simulink model "DisplayModel_Step2_start"  (R2013b)
settings: Solver=FixedStepDiscrete  StartTime=0.0  StopTime=10.0  FixedStep=0.2  RelTol=1e-3
undefined symbols (not defined in the file): sigbuilder_block
libraries: simulink x6
settings Model: CovHTMLOptions=-sRT=1 -aTS=1 -bRG=1 -bTC=1 -hTR=0 -nFC=0 -scm=1 -bcm=1 -xEv=0  Creator=siddhars  LastModifiedBy=rruff
settings OptimizationCC: ExpressionDepthLimit=2147483647
settings DebuggingCC: StateNameClashWarn=warning

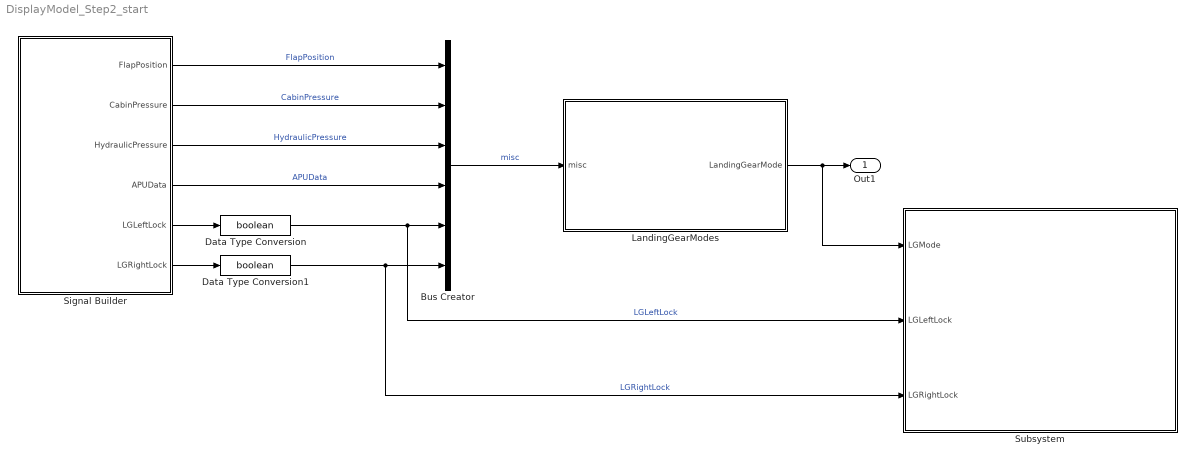
== system DisplayModel_Step2_start ==
  Bus Creator : BusCreator  Inputs=6  OutDataTypeStr=Bus: MiscData
  Data Type Conversion : DataTypeConversion  OutDataTypeStr=boolean
  Data Type Conversion1 : DataTypeConversion  OutDataTypeStr=boolean
  LandingGearModes : Stateflow chart  TreatAsAtomicUnit=on
  Signal Builder : Subsystem  Tag=STV Subsys  LoadFcn=sigbuilder_block('load');  StartFcn=sigbuilder_block('start');  StopFcn=sigbuilder_block('stop');  ClipboardFcn=sigbuilder_block('clipboard');  mask(Sigbuilder block){}
      mask help: Simulink:masks:SigbuilderBlock_MD
      mask init:
      | if ~strcmp(get_param(bdroot(gcbh),'SimulationStatus'),'stopped') tuvar = sigbuilder_block('maskInit'); end
      settings: CopyFcn=sigbuilder_block('copy');  DeleteFcn=sigbuilder_block('delete');  ModelCloseFcn=sigbuilder_block('modelClose');  PreSaveFcn=sigbuilder_block('preSave');  PauseFcn=sigbuilder_block('pause');  ContinueFcn=sigbuilder_block('continue');  NameChangeFcn=sigbuilder_block('namechange');  OpenFcn=sigbuilder_block('open',[43.5 185.25 692.25 402.75 ]);  CloseFcn=sigbuilder_block('close');
      mask Display: plot(0, 0, 100, 100,[2, 2, 32, 32, 2], [68, 8, 8, 68, 68],[32, 2], [38, 38], [32, 19, 2],[53, 60, 44], [32, 17, 17, 2],[16, 16, 31, 31]);txt = getActiveGroup(gcbh);text(2, 100, txt,'verticalAlignment', 'top');
  Subsystem : Subsystem
  Out1 : Outport
  wires:
  LandingGearModes/1(LandingGearMode) -> Subsystem/1(LGMode), Out1/1
  Signal Builder/6(LGRightLock) -> Data Type Conversion1/1
  Signal Builder/5(LGLeftLock) -> Data Type Conversion/1
  Data Type Conversion1/1 -> Subsystem/3(LGRightLock), Bus Creator/6  "LGRightLock"
  Data Type Conversion/1 -> Subsystem/2(LGLeftLock), Bus Creator/5  "LGLeftLock"
  Signal Builder/1(FlapPosition) -> Bus Creator/1  "FlapPosition"
  Signal Builder/3(HydraulicPressure) -> Bus Creator/3  "HydraulicPressure"
  Signal Builder/4(APUData) -> Bus Creator/4  "APUData"
  Signal Builder/2(CabinPressure) -> Bus Creator/2  "CabinPressure"
  Bus Creator/1 -> LandingGearModes/1(misc)  "misc"

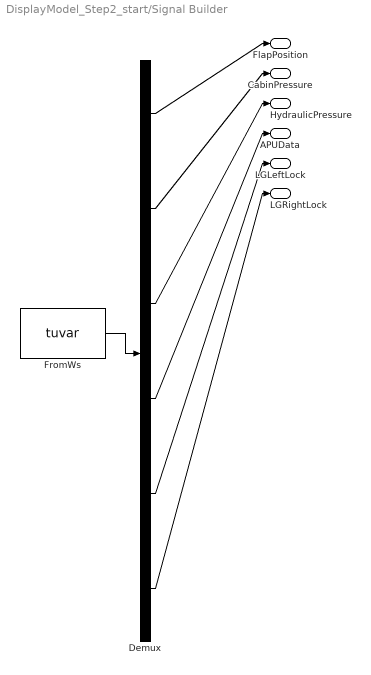
== system DisplayModel_Step2_start/Signal Builder ==
  Demux : Demux  Tag=STV Demux  Outputs=6
  FromWs : FromWorkspace  Tag=STV FromWs  VariableName=tuvar  SampleTime=0
      SigBuilderData=|
      | common.afterFinalStr = 'Extrapolate'
      | common.sampleTime = 0
      | dataSet(1).timeRange = [0 10]
      | dataSet(1).name = 'BothOn'
      | dataSet(2).timeRange = [0 10]
      | dataSet(2).name = 'OneOnA'
      | dataSet(3).timeRange = [0 10]
      | dataSet(3).name = 'OneOnB'
      | dataSet(4).timeRange = [0 10]
      | dataSet(4).name = 'BothOFF'
      | sbobj.Groups(1).Name = 'BothOn'
      | sbobj.Groups(1).Signals(1).Name = 'FlapPosition'
      | sbobj.Groups(1).Signals(1).XData = [0 10]
      | sbobj.Groups(1).Signals(1).YData = [0 0]
      | sbobj.Groups(1).Signals(2).Name = 'CabinPressure'
      | sbobj.Groups(1).Signals(2).XData = [0 10]
      | sbobj.Groups(1).Signals(2).YData = [0 0]
      | sbobj.Groups(1).Signals(3).Name = 'HydraulicPressure'
      | sbobj.Groups(1).Signals(3).XData = [0 10]
      | sbobj.Groups(1).Signals(3).YData = [0 0]
      | sbobj.Groups(1).Signals(4).Name = 'APUData'
      | sbobj.Groups(1).Signals(4).XData = [0 10]
      | sbobj.Groups(1).Signals(4).YData = [0 0]
      | sbobj.Groups(1).Signals(5).Name = 'LGLeftLock'
      | sbobj.Groups(1).Signals(5).XData = [0 1.74 6.62 10]
      | sbobj.Groups(1).Signals(5).YData = [1 1 1 1]
      | sbobj.Groups(1).Signals(6).Name = 'LGRightLock'
      | sbobj.Groups(1).Signals(6).XData = [0 3.36 7.8 10]
      | sbobj.Groups(1).Signals(6).YData = [1 1 1 1]
      | sbobj.Groups(2).Name = 'OneOnA'
      | sbobj.Groups(2).Signals(1).Name = 'FlapPosition'
      | sbobj.Groups(2).Signals(1).XData = [0 10]
      | sbobj.Groups(2).Signals(1).YData = [0 0]
      | sbobj.Groups(2).Signals(2).Name = 'CabinPressure'
      | sbobj.Groups(2).Signals(2).XData = [0 10]
      | sbobj.Groups(2).Signals(2).YData = [0 0]
      | sbobj.Groups(2).Signals(3).Name = 'HydraulicPressure'
      | sbobj.Groups(2).Signals(3).XData = [0 10]
      | sbobj.Groups(2).Signals(3).YData = [0 0]
      | sbobj.Groups(2).Signals(4).Name = 'APUData'
      | sbobj.Groups(2).Signals(4).XData = [0 10]
      | sbobj.Groups(2).Signals(4).YData = [0 0]
      | sbobj.Groups(2).Signals(5).Name = 'LGLeftLock'
      | sbobj.Groups(2).Signals(5).XData = [0 5.02 5.02 10]
      | sbobj.Groups(2).Signals(5).YData = [1 1 0 0]
      | sbobj.Groups(2).Signals(6).Name = 'LGRightLock'
      | sbobj.Groups(2).Signals(6).XData = [0 5.02 5.02 10]
      | sbobj.Groups(2).Signals(6).YData = [0 0 1 1]
      | sbobj.Groups(3).Name = 'OneOnB'
      | sbobj.Groups(3).Signals(1).Name = 'FlapPosition'
      | sbobj.Groups(3).Signals(1).XData = [0 10]
      | sbobj.Groups(3).Signals(1).YData = [0 0]
      | sbobj.Groups(3).Signals(2).Name = 'CabinPressure'
      | sbobj.Groups(3).Signals(2).XData = [0 10]
      | sbobj.Groups(3).Signals(2).YData = [0 0]
      | sbobj.Groups(3).Signals(3).Name = 'HydraulicPressure'
      | sbobj.Groups(3).Signals(3).XData = [0 10]
      | sbobj.Groups(3).Signals(3).YData = [0 0]
      | sbobj.Groups(3).Signals(4).Name = 'APUData'
      | sbobj.Groups(3).Signals(4).XData = [0 10]
      | sbobj.Groups(3).Signals(4).YData = [0 0]
      | sbobj.Groups(3).Signals(5).Name = 'LGLeftLock'
      | sbobj.Groups(3).Signals(5).XData = [0 5.02 5.02 10]
      | sbobj.Groups(3).Signals(5).YData = [0 0 1 1]
      | sbobj.Groups(3).Signals(6).Name = 'LGRightLock'
      | sbobj.Groups(3).Signals(6).XData = [0 5.02 5.02 10]
      | sbobj.Groups(3).Signals(6).YData = [1 1 0 0]
      | sbobj.Groups(4).Name = 'BothOFF'
      | sbobj.Groups(4).Signals(1).Name = 'FlapPosition'
      | sbobj.Groups(4).Signals(1).XData = [0 10]
      | sbobj.Groups(4).Signals(1).YData = [0 0]
      | sbobj.Groups(4).Signals(2).Name = 'CabinPressure'
      | sbobj.Groups(4).Signals(2).XData = [0 10]
      | sbobj.Groups(4).Signals(2).YData = [0 0]
      | sbobj.Groups(4).Signals(3).Name = 'HydraulicPressure'
      | sbobj.Groups(4).Signals(3).XData = [0 10]
      | sbobj.Groups(4).Signals(3).YData = [0 0]
      | sbobj.Groups(4).Signals(4).Name = 'APUData'
      | sbobj.Groups(4).Signals(4).XData = [0 10]
      | sbobj.Groups(4).Signals(4).YData = [0 0]
      | sbobj.Groups(4).Signals(5).Name = 'LGLeftLock'
      | sbobj.Groups(4).Signals(5).XData = [0 10]
      | sbobj.Groups(4).Signals(5).YData = [0 0]
      | sbobj.Groups(4).Signals(6).Name = 'LGRightLock'
      | sbobj.Groups(4).Signals(6).XData = [0 10]
      | sbobj.Groups(4).Signals(6).YData = [0 0]
  FlapPosition : Outport  Tag=STV Outport
  CabinPressure : Outport  Tag=STV Outport  Port=2
  HydraulicPressure : Outport  Tag=STV Outport  Port=3
  APUData : Outport  Tag=STV Outport  Port=4
  LGLeftLock : Outport  Tag=STV Outport  Port=5
  LGRightLock : Outport  Tag=STV Outport  Port=6
  wires:
  FromWs/1 -> Demux/1
  Demux/1 -> FlapPosition/1
  Demux/2 -> CabinPressure/1
  Demux/3 -> HydraulicPressure/1
  Demux/4 -> APUData/1
  Demux/5 -> LGLeftLock/1
  Demux/6 -> LGRightLock/1

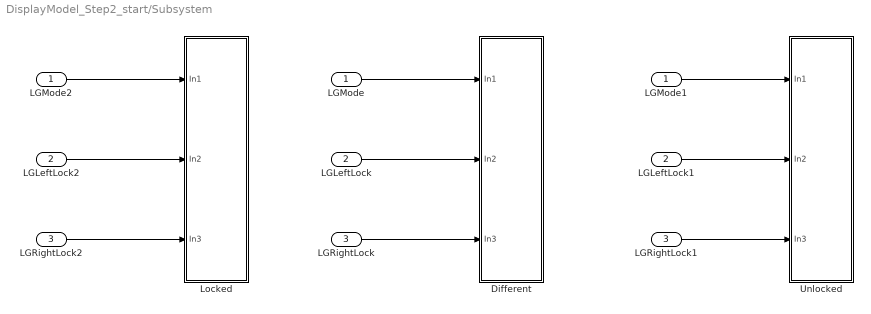
== system DisplayModel_Step2_start/Subsystem ==
  LGMode : Inport
  LGLeftLock : Inport  Port=2
  LGRightLock : Inport  Port=3
  Different : Subsystem
  LGLeftLock1 : InportShadow  Port=2
  LGLeftLock2 : InportShadow  Port=2
  LGMode1 : InportShadow
  LGMode2 : InportShadow
  LGRightLock1 : InportShadow  Port=3
  LGRightLock2 : InportShadow  Port=3
  Locked : Subsystem
  Unlocked : Subsystem
  wires:
  LGLeftLock/1 -> Different/2(In2)
  LGLeftLock1/1 -> Unlocked/2(In2)
  LGMode2/1 -> Locked/1(In1)
  LGRightLock2/1 -> Locked/3(In3)
  LGMode1/1 -> Unlocked/1(In1)
  LGRightLock/1 -> Different/3(In3)
  LGMode/1 -> Different/1(In1)
  LGLeftLock2/1 -> Locked/2(In2)
  LGRightLock1/1 -> Unlocked/3(In3)

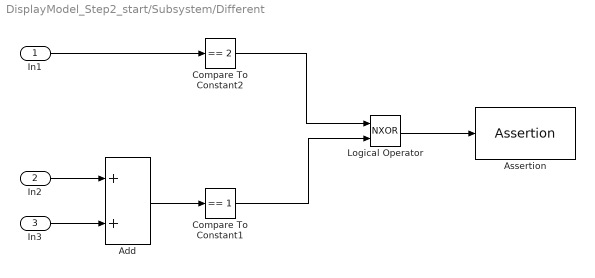
== system DisplayModel_Step2_start/Subsystem/Different ==
  In1 : Inport
  In2 : Inport  Port=2
  In3 : Inport  Port=3
  Add : Sum
  Assertion : Assertion  Enabled=off
  Compare To Constant1 : simulink/Logic and Bit Operations/Compare To Constant  relop===  const=1  OutDataTypeStr=uint8
  Compare To Constant2 : simulink/Logic and Bit Operations/Compare To Constant  relop===  const=2  OutDataTypeStr=boolean
  Logical Operator : Logic  Operator=NXOR  AllPortsSameDT=off  OutDataTypeStr=boolean
  wires:
  Logical Operator/1 -> Assertion/1
  Compare To Constant2/1 -> Logical Operator/1
  In1/1 -> Compare To Constant2/1
  Add/1 -> Compare To Constant1/1
  Compare To Constant1/1 -> Logical Operator/2
  In2/1 -> Add/1
  In3/1 -> Add/2

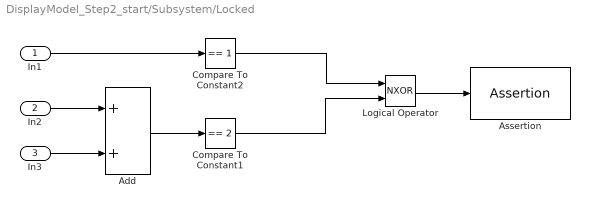
== system DisplayModel_Step2_start/Subsystem/Locked ==
  In1 : Inport
  In2 : Inport  Port=2
  In3 : Inport  Port=3
  Add : Sum
  Assertion : Assertion  Enabled=off
  Compare To Constant1 : simulink/Logic and Bit Operations/Compare To Constant  relop===  const=2  OutDataTypeStr=uint8
  Compare To Constant2 : simulink/Logic and Bit Operations/Compare To Constant  relop===  const=1  OutDataTypeStr=uint8
  Logical Operator : Logic  Operator=NXOR  AllPortsSameDT=off  OutDataTypeStr=boolean
  wires:
  Add/1 -> Compare To Constant1/1
  Logical Operator/1 -> Assertion/1
  Compare To Constant1/1 -> Logical Operator/2
  In2/1 -> Add/1
  In3/1 -> Add/2
  In1/1 -> Compare To Constant2/1
  Compare To Constant2/1 -> Logical Operator/1

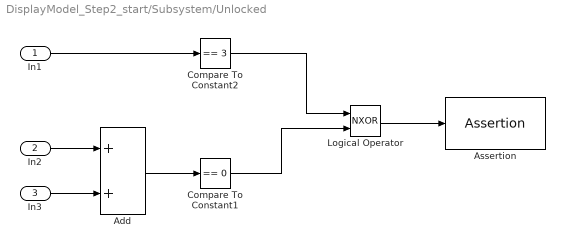
== system DisplayModel_Step2_start/Subsystem/Unlocked ==
  In1 : Inport
  In2 : Inport  Port=2
  In3 : Inport  Port=3
  Add : Sum
  Assertion : Assertion  Enabled=off
  Compare To Constant1 : simulink/Logic and Bit Operations/Compare To Constant  relop===  const=0  OutDataTypeStr=uint8
  Compare To Constant2 : simulink/Logic and Bit Operations/Compare To Constant  relop===  const=3  OutDataTypeStr=uint8
  Logical Operator : Logic  Operator=NXOR  AllPortsSameDT=off  OutDataTypeStr=boolean
  wires:
  Logical Operator/1 -> Assertion/1
  Compare To Constant2/1 -> Logical Operator/1
  In1/1 -> Compare To Constant2/1
  Add/1 -> Compare To Constant1/1
  Compare To Constant1/1 -> Logical Operator/2
  In2/1 -> Add/1
  In3/1 -> Add/2

== stateflow chart DisplayModel_Step2_start/LandingGearModes ==
  state LeftLock [parallel]
    settings: executionOrder=1
    state Unlocked
    state Locked
    (default) -> (junction 122)
    (junction 122) -> LeftLock.Unlocked [order 2]
    (junction 122) -> LeftLock.Locked [order 1] : [misc.LGLeftLock]
    LeftLock.Locked -> LeftLock.Unlocked : [~misc.LGLeftLock]
    LeftLock.Unlocked -> LeftLock.Locked : [misc.LGLeftLock]
  state RightLock [parallel]
    settings: executionOrder=2
    state Unlocked
    state Locked
    (default) -> (junction 136)
    (junction 136) -> RightLock.Unlocked [order 2]
    (junction 136) -> RightLock.Locked [order 1] : [misc.LGRightLock]
    RightLock.Locked -> RightLock.Unlocked : [~misc.LGRightLock]
    RightLock.Unlocked -> RightLock.Locked : [misc.LGRightLock]
  state WarningModes [parallel]
    settings: executionOrder=3
    state BothLocked
      entry:
      LandingGearMode = 1;
    state BothUnLocked
      entry:
      LandingGearMode = 3;
    state OnlyOneLocked
      entry:
      LandingGearMode = 2;
    (default) -> (junction 102)
    (junction 102) -> BothLocked [order 1] : [in(LeftLock.Locked) &&...
        | in(RightLock.Locked)]
    (junction 102) -> BothUnLocked [order 3]
    (junction 102) -> OnlyOneLocked [order 2] : [in(LeftLock.Unlocked) ||...
        | in(RightLock.Unlocked)]
    BothUnLocked -> OnlyOneLocked [order 1] : [in(LeftLock.Locked) ||...
        | in(RightLock.Locked)]
    OnlyOneLocked -> BothLocked [order 2] : [in(LeftLock.Locked) &&...
        | in(RightLock.Locked)]
    OnlyOneLocked -> BothUnLocked [order 1] : [in(LeftLock.Unlocked) &&...
        | in(RightLock.Unlocked)]
    BothLocked -> OnlyOneLocked [order 1] : [in(LeftLock.Unlocked) ||...
        | in(RightLock.Unlocked)]
    BothLocked -> BothUnLocked [order 2] : [in(LeftLock.Unlocked) &&...
        | in(RightLock.Unlocked)]
    BothUnLocked -> BothLocked [order 2] : [in(LeftLock.Locked) &&...
        | in(RightLock.Locked)]
  data: misc input Bus: MiscData; LandingGearMode output double size=1
